simulink model "Trajectory_Planning_with_Kinematics"  (R2019a)
settings: Solver=FixedStepAuto  StartTime=0.0  StopTime=10  FixedStep=0.01  RelTol=1e-3
libraries: mobileRoboticsLib x1
settings Model: Creator=HP  LastModifiedBy=chute

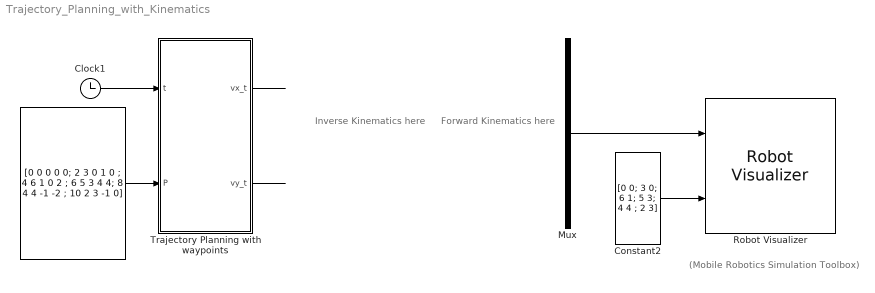
== system Trajectory_Planning_with_Kinematics ==
  note: (Mobile Robotics Simulation Toolbox)
  note: Forward
      | Kinematics
      | here
  note: Inverse
      | Kinematics
      | here
  " " : Constant  Value=[0 0 0 0 0; 2 3 0 1 0 ; 4 6 1 0 2 ; 6 5 3 4 4; 8 4 4 -1 -2 ; 10 2 3 -1 0]  VectorParams1D=off  SampleTime=-1
  Clock1 : Clock
  Constant2 : Constant  Value=[0 0; 3 0; 6 1; 5 3; 4 4 ; 2 3]
  Mux : Mux  Inputs=3
  "Robot Visualizer " : mobileRoboticsLib/Environments/Robot Visualizer  robotRadius=0  showTrajectory=on  hasWaypoints=on  hasLidar=off  sensorOffset=[ 0, 0 ]  scanAngles=[ -pi/4, 0, pi/4 ]  hasObjDetector=off  objDetectorOffset=[ 0, 0 ]  objDetectorAngle=0  objDetectorFOV=pi/4  objDetectorMaxRange=5  objectColors=[ 1, 0, 0; 0, 1, 0; 0, 0, 1 ]  objectMarkers=s
  Trajectory Planning with waypoints : MATLAB Function  TreatAsAtomicUnit=on
  wires:
  ? -> Mux/1
  ? -> Mux/2
  ? -> Mux/3
  ? -> ?
  ? -> ?
  Mux/1 -> "Robot Visualizer "/1
  Clock1/1 -> Trajectory Planning with waypoints/1(t)
  " "/1 -> Trajectory Planning with waypoints/2(P)
  Trajectory Planning with waypoints/1(vx_t) -> ?
  Trajectory Planning with waypoints/2(vy_t) -> ?
  Constant2/1 -> "Robot Visualizer "/2

== matlab function Trajectory_Planning_with_Kinematics/Trajectory Planning with waypoints ==
  data: t input; vx_t output; vy_t output; P input
function [vx_t,vy_t] = fcn(t,P)
%% Quy hoach quy dao
k = size(P,1)-1;                                        % So giai doan chay, i diem thi i-1 giai doan
ai = zeros(k,8);                                        % Ma tran K*8 luu cac gia tri a0-a4 cua X,Y
for i=1:k
    ai(i,:) = Trajectory_Planning(P(i,:),P(i+1,:));     % Tinh gia tri a0-a4 doi voi tung diem P(x,y)
end
%% Xuat quy dao
ti = P(2,1);                                            % Thoi gian lay mau giua 2 diem
if(t<P(k+1,1))
    j = floor(t/ti)+1;                                  % Xac dinh giai doan hien tai cua quy dao
    vx_t = ai(j,2) + 2*ai(j,3)*t + 3*ai(j,4)*t^2;
    vy_t = ai(j,6) + 2*ai(j,7)*t + 3*ai(j,8)*t^2;
else
    vx_t = P(k+1,4);
    vy_t = P(k+1,5);
end
end
